simulink model "Ej10"  (R2025a)
settings: Solver=VariableStepAuto  StartTime=0.0  StopTime=10.0  RelTol=1e-3
libraries: dspsrcs4 x10, commrandsrc3 x4, dspfdesign x2
settings Model: Creator=Henry  LastModifiedBy=Henry

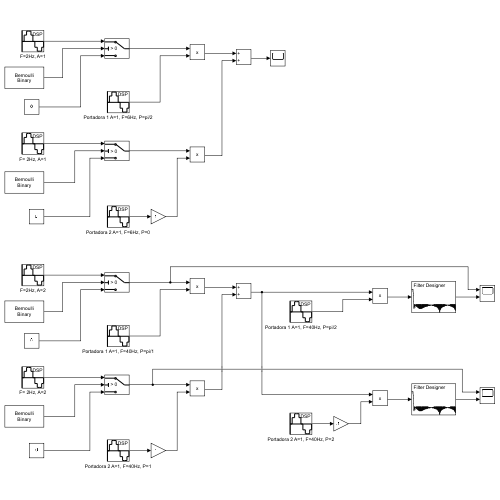
[thumbnail: Simulink's stored preview of the top-level diagram]
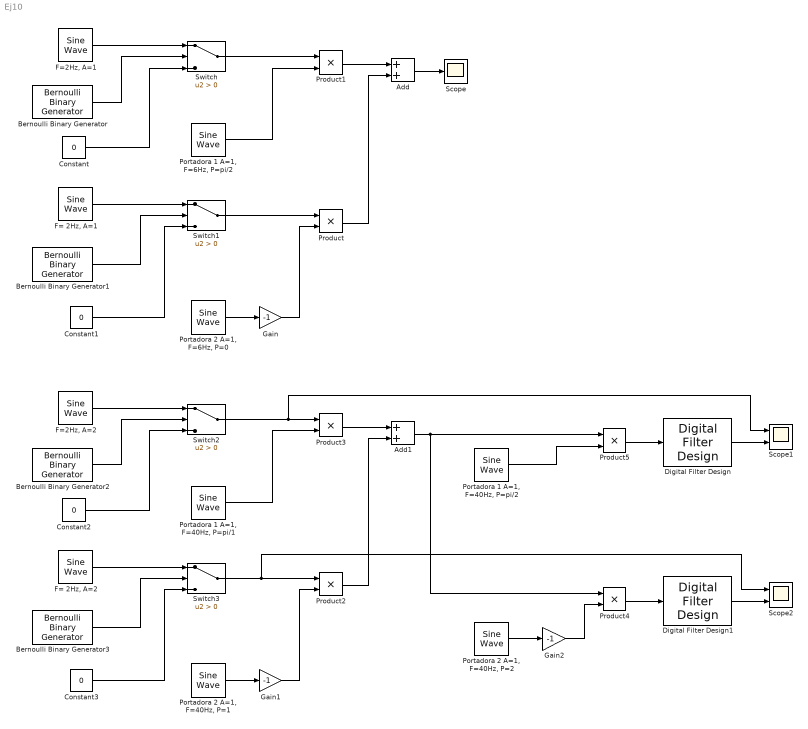
== system Ej10 ==
  Add : Sum
  Add1 : Sum
  Bernoulli Binary Generator{,1..3} (4 alike) : commrandsrc3/Bernoulli Binary Generator  ProbabilityOfZero=0.5  SeedSource=Auto  Seed=0  SampleTime=1  SamplesPerFrame=1  OutputDataType=double  SimulateUsing=Interpreted execution
  Constant{,1..3} (4 alike) : Constant  Value=0
  Digital Filter Design : dspfdesign/Digital Filter Design  mwdsp_browser_bugfix_var=off
  Digital Filter Design1 : dspfdesign/Digital Filter Design  mwdsp_browser_bugfix_var=off
  "F= 2Hz, A=1" : dspsrcs4/Sine Wave  Amplitude=1  Frequency=2  Phase=0  SampleMode=Discrete  OutComplex=Real  CompMethod=Trigonometric fcn  TableSize=Speed  SampleTime=1/1000  SamplesPerFrame=1  ResetState=Restart at time zero  OutputFrames=off  dataType=double  wordLen=16  udDataType=sfix(16)  fracBitsMode=Best precision  numFracBits=15  OutDataTypeStr=double  LastOutDataTypeStr=double
  "F= 2Hz, A=2" : dspsrcs4/Sine Wave  Amplitude=1  Frequency=2  Phase=0  SampleMode=Discrete  OutComplex=Real  CompMethod=Trigonometric fcn  TableSize=Speed  SampleTime=1/1000  SamplesPerFrame=1  ResetState=Restart at time zero  OutputFrames=off  dataType=double  wordLen=16  udDataType=sfix(16)  fracBitsMode=Best precision  numFracBits=15  OutDataTypeStr=double  LastOutDataTypeStr=double
  "F=2Hz, A=1" : dspsrcs4/Sine Wave  Amplitude=1  Frequency=2  Phase=0  SampleMode=Discrete  OutComplex=Real  CompMethod=Trigonometric fcn  TableSize=Speed  SampleTime=1/1000  SamplesPerFrame=1  ResetState=Restart at time zero  OutputFrames=off  dataType=double  wordLen=16  udDataType=sfix(16)  fracBitsMode=Best precision  numFracBits=15  OutDataTypeStr=double  LastOutDataTypeStr=double
  "F=2Hz, A=2" : dspsrcs4/Sine Wave  Amplitude=1  Frequency=2  Phase=0  SampleMode=Discrete  OutComplex=Real  CompMethod=Trigonometric fcn  TableSize=Speed  SampleTime=1/1000  SamplesPerFrame=1  ResetState=Restart at time zero  OutputFrames=off  dataType=double  wordLen=16  udDataType=sfix(16)  fracBitsMode=Best precision  numFracBits=15  OutDataTypeStr=double  LastOutDataTypeStr=double
  Gain : Gain  Gain=-1
  Gain1 : Gain  Gain=-1
  Gain2 : Gain  Gain=-1
  "Portadora 1 A=1, F=40Hz, P=pi/1" : dspsrcs4/Sine Wave  Amplitude=1  Frequency=40  Phase=pi/2  SampleMode=Discrete  OutComplex=Real  CompMethod=Trigonometric fcn  TableSize=Speed  SampleTime=1/1000  SamplesPerFrame=1  ResetState=Restart at time zero  OutputFrames=off  dataType=double  wordLen=16  udDataType=sfix(16)  fracBitsMode=Best precision  numFracBits=15  OutDataTypeStr=double  LastOutDataTypeStr=double
  "Portadora 1 A=1, F=40Hz, P=pi/2" : dspsrcs4/Sine Wave  Amplitude=1  Frequency=40  Phase=pi/2  SampleMode=Discrete  OutComplex=Real  CompMethod=Trigonometric fcn  TableSize=Speed  SampleTime=1/1000  SamplesPerFrame=1  ResetState=Restart at time zero  OutputFrames=off  dataType=double  wordLen=16  udDataType=sfix(16)  fracBitsMode=Best precision  numFracBits=15  OutDataTypeStr=double  LastOutDataTypeStr=double
  "Portadora 1 A=1, F=6Hz, P=pi/2" : dspsrcs4/Sine Wave  Amplitude=1  Frequency=6  Phase=pi/2  SampleMode=Discrete  OutComplex=Real  CompMethod=Trigonometric fcn  TableSize=Speed  SampleTime=1/1000  SamplesPerFrame=1  ResetState=Restart at time zero  OutputFrames=off  dataType=double  wordLen=16  udDataType=sfix(16)  fracBitsMode=Best precision  numFracBits=15  OutDataTypeStr=double  LastOutDataTypeStr=double
  "Portadora 2 A=1, F=40Hz, P=1" : dspsrcs4/Sine Wave  Amplitude=1  Frequency=40  Phase=0  SampleMode=Discrete  OutComplex=Real  CompMethod=Trigonometric fcn  TableSize=Speed  SampleTime=1/1000  SamplesPerFrame=1  ResetState=Restart at time zero  OutputFrames=off  dataType=double  wordLen=16  udDataType=sfix(16)  fracBitsMode=Best precision  numFracBits=15  OutDataTypeStr=double  LastOutDataTypeStr=double
  "Portadora 2 A=1, F=40Hz, P=2" : dspsrcs4/Sine Wave  Amplitude=1  Frequency=40  Phase=0  SampleMode=Discrete  OutComplex=Real  CompMethod=Trigonometric fcn  TableSize=Speed  SampleTime=1/1000  SamplesPerFrame=1  ResetState=Restart at time zero  OutputFrames=off  dataType=double  wordLen=16  udDataType=sfix(16)  fracBitsMode=Best precision  numFracBits=15  OutDataTypeStr=double  LastOutDataTypeStr=double
  "Portadora 2 A=1, F=6Hz, P=0" : dspsrcs4/Sine Wave  Amplitude=1  Frequency=6  Phase=0  SampleMode=Discrete  OutComplex=Real  CompMethod=Trigonometric fcn  TableSize=Speed  SampleTime=1/1000  SamplesPerFrame=1  ResetState=Restart at time zero  OutputFrames=off  dataType=double  wordLen=16  udDataType=sfix(16)  fracBitsMode=Best precision  numFracBits=15  OutDataTypeStr=double  LastOutDataTypeStr=double
  Product{,1..5} (6 alike) : Product
  Scope : Scope
      settings: ActiveDisplayYMinimum=-1  ActiveDisplayYMaximum=1
  Scope1 : Scope  NumInputPorts=2
      settings: ActiveDisplayYMinimum=-1.25  ActiveDisplayYMaximum=1.25
  Scope2 : Scope  NumInputPorts=2
      settings: ActiveDisplayYMinimum=-1.25  ActiveDisplayYMaximum=1.25  DataLoggingVariableName=ScopeData2
  Switch{,1..3} (4 alike) : Switch  Criteria=u2 > Threshold  SaturateOnIntegerOverflow=off  InputSameDT=off
  wires:
  Bernoulli Binary Generator/1 -> Switch/2
  "F=2Hz, A=1"/1 -> Switch/1
  Constant/1 -> Switch/3
  "F= 2Hz, A=1"/1 -> Switch1/1
  Bernoulli Binary Generator1/1 -> Switch1/2
  Constant1/1 -> Switch1/3
  "Portadora 2 A=1, F=6Hz, P=0"/1 -> Gain/1
  Switch1/1 -> Product/1
  Gain/1 -> Product/2
  Switch/1 -> Product1/1
  "Portadora 1 A=1, F=6Hz, P=pi/2"/1 -> Product1/2
  Product1/1 -> Add/1
  Product/1 -> Add/2
  Add/1 -> Scope/1
  Product2/1 -> Add1/2
  Product3/1 -> Add1/1
  Constant3/1 -> Switch3/3
  "Portadora 1 A=1, F=40Hz, P=pi/1"/1 -> Product3/2
  Switch2/1 -> Scope1/1, Product3/1
  Bernoulli Binary Generator3/1 -> Switch3/2
  Switch3/1 -> Scope2/1, Product2/1
  Gain1/1 -> Product2/2
  Constant2/1 -> Switch2/3
  Bernoulli Binary Generator2/1 -> Switch2/2
  "Portadora 2 A=1, F=40Hz, P=1"/1 -> Gain1/1
  "F=2Hz, A=2"/1 -> Switch2/1
  "F= 2Hz, A=2"/1 -> Switch3/1
  "Portadora 2 A=1, F=40Hz, P=2"/1 -> Gain2/1
  "Portadora 1 A=1, F=40Hz, P=pi/2"/1 -> Product5/2
  Gain2/1 -> Product4/2
  Add1/1 -> Product4/1, Product5/1
  Product5/1 -> Digital Filter Design/1
  Product4/1 -> Digital Filter Design1/1
  Digital Filter Design/1 -> Scope1/2
  Digital Filter Design1/1 -> Scope2/2
